simulink model "sim4_221036"  (R2022b)
settings: Solver=VariableStepAuto  StartTime=0.0  StopTime=10.0  RelTol=1e-3
settings Model: Creator=Administrator  LastModifiedBy=Administrator

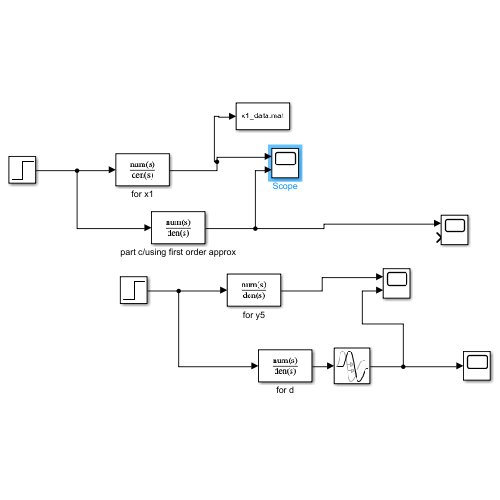
[thumbnail: Simulink's stored preview of the top-level diagram]
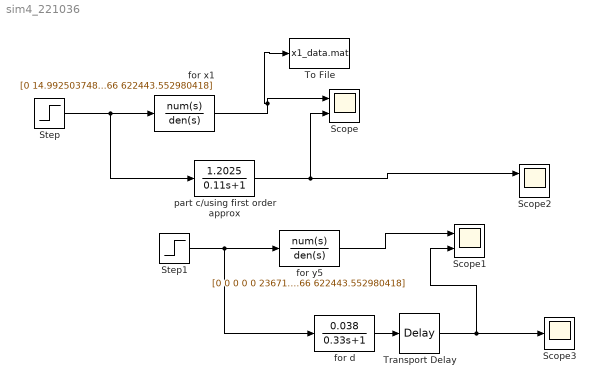
== system sim4_221036 ==
  Scope : Scope  NumInputPorts=2
  Scope1 : Scope  NumInputPorts=2
  Scope2 : Scope  NumInputPorts=2
  Scope3 : Scope
  Step : Step  Time=0  After=0.05  SampleTime=0
  Step1 : Step  Time=0  After=0.05  SampleTime=0
  To File : ToFile  Filename=x1_data.mat  SampleTime=0.0001
  Transport Delay : TransportDelay  DelayTime=0.54
  for d : TransferFcn  Numerator=[0.038]  Denominator=[0.33 1]
  for x1 : TransferFcn  Numerator=[0 14.9925037481259 1168.83087691537 30127.2864710626 286369.331639521 748465.401895939]  Denominator=[1 97.4512743628186 3439.06008015483 53009.1964418138 335907.992485066 622443.552980418]
  for y5 : TransferFcn  Numerator=[0 0 0 0 0 23671.2314636657]  Denominator="[1\t97.4512743628186\t3439.06008015483\t53009.1964418138\t335907.992485066\t622443.552980418]"
  part c/using first order approx : TransferFcn  Numerator=[1.2025]  Denominator=[0.11 1]
  wires:
  Step/1 -> part c/using first order approx/1, for x1/1
  for x1/1 -> To File/1, Scope/1
  for y5/1 -> Scope1/1
  Step1/1 -> for d/1, for y5/1
  part c/using first order approx/1 -> Scope/2, Scope2/1
  Transport Delay/1 -> Scope1/2, Scope3/1
  for d/1 -> Transport Delay/1
